simulink model "ammclib_gdflib_iir2_s32k14x"  (Simulink 9.0)
settings: Solver=FixedStepDiscrete  StartTime=0.0  StopTime=5  FixedStep=0.001  RelTol=1e-3  EnableMultiTasking=on
PostLoadFcn:
  | ammclib_gdflib_iir2_s32k14x_params()
InitFcn:
  | mbd_s32k_consistency_checks(bdroot(gcs));
undefined symbols (not defined in the file or in its folder): LQFP
libraries: ammclib_bam_s32k14x x7, mbd_s32k1xx_ec_toolbox x2, simulink x1
Description:
  | This model tests the AMMCLIB GDFLIB IIR2 blocks
  | 
  | Validation:
  | - Run the model in Simulation and check if the results look like the ones shown in the scope capture
  | - Open Freemaster (ammclib_gdflib_iir2_s32k14x.pmp) and compare the HW results against the Simulated ones
CloseFcn:
  | clear all;
settings Model: Creator=NXP MBDT Team  LastModifiedBy=nxf35172
settings DataIOCC: ExternalInput=off  InitialState=off  LimitDataPoints=on  SaveOutput=off  SignalLogging=off  SaveTime=off
settings OptimizationCC: DefaultParameterBehavior=Inlined  LifeSpan=1
settings DebuggingCC: SolverPrmCheckMsg=warning  InheritedTsInSrcMsg=none  SingleTaskRateTransMsg=error  ParameterPrecisionLossMsg=none  UnconnectedInputMsg=error  UnconnectedOutputMsg=error  UnconnectedLineMsg=error  AllowSymbolicDim=off  UnknownTsInhSupMsg=error  StateNameClashWarn=warning
settings HardwareCC: ProdLargestAtomicInteger=Long  ProdLargestAtomicFloat=Double  ProdEndianess=LittleEndian  ProdHWDeviceType=ARM Compatible->ARM Cortex
settings SFSimCC: MATLABDynamicMemAlloc=off
settings RTWCC: SystemTargetFile=mbd_s32k.tlc  MakeCommand=mbd_s32k_make_rtw COPY_MDLREF_INCLUDES=0  TemplateMakefile=mbd_s32k.tmf  Description=Model Based Design Toolbox S32K14x Code Generation Target
settings CodeAppCC: IgnoreCustomStorageClasses=off
settings STFCustomTargetCC: CombineOutputUpdateFcns=on  ERTCustomFileBanners=on  SupportContinuousTime=off  SupportNonInlinedSFcns=off  RemoveResetFunc=on  MATLABClassNameForMDSCustomization=Simulink.SoftwareTarget.ERTCustomization  GRTInterface=off  SystemTargetFile=mbd_s32k14.tlc
settings ERTTargetCC: MultiwordLength=2048  ParMdlRefBuildCompliant=off  CompOptLevelCompliant=off  ConcurrentExecutionCompliant=off  ModelStepFunctionPrototypeControlCompliant=off  CPPClassGenCompliant=off  UseToolchainInfoCompliant=off  InlinedParameterPlacement=NonHierarchical  ERTCustomFileTemplate=example_file_process.tlc  ConvertIfToSwitch=off  SuppressUnreachableDefaultCases=off  MaxIdInt32=IIR2X_int32_T  MaxIdUint32=IIR2X_uint32_T  MaxIdInt16=IIR2X_int16_T  MaxIdUint16=IIR2X_uint16_T  MaxIdInt8=IIR2X_int8_T  MaxIdUint8=IIR2X_uint8_T

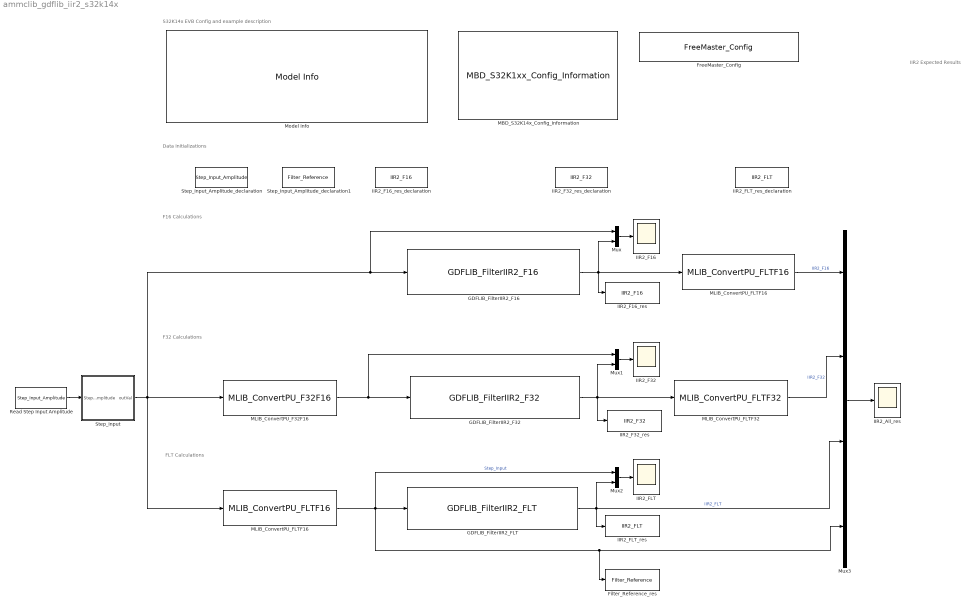
== system ammclib_gdflib_iir2_s32k14x ==
  note: IIR2 Expected Results
  note: S32K14x EVB Config and example description
  note: Data Initializations
  note: F16 Calculations
  note: F32 Calculations
  note: FLT Calculations
  Filter_Reference_res : DataStoreWrite  DataStoreName=Filter_Reference
  FreeMaster_Config : mbd_s32k1xx_ec_toolbox/Utility Blocks/FreeMaster_Config  interface=LPUART1  baudrate=115200  rxd=PTC6: [LPUART1_RX | Receive]  txd=PTC7: [LPUART1_TX | Transmit]  mode=Short Interrupt  isr_prio=15  show_adv_opts=off  use_scope=on  max_scope_vars=8  use_recorder=on  max_rec_vars=8  rec_buff_size=1024  rec_timebase=0 milliseconds  comm_buffer_size_auto=on  comm_buffer_size=255  comm_rqueue_size_default=on  comm_rqueue_size=32
  GDFLIB_FilterIIR2_F16 : ammclib_bam_s32k14x/GDFLIB/bam_f16/GDFLIB_FilterIIR2_F16  f16B0=f16B0  f16B1=f16B1  f16B2=f16B2  f16A1=f16A1  f16A2=f16A2
  GDFLIB_FilterIIR2_F32 : ammclib_bam_s32k14x/GDFLIB/bam_f32/GDFLIB_FilterIIR2_F32  f32B0=f32B0  f32B1=f32B1  f32B2=f32B2  f32A1=f32A1  f32A2=f32A2
  GDFLIB_FilterIIR2_FLT : ammclib_bam_s32k14x/GDFLIB/bam_flt/GDFLIB_FilterIIR2_FLT  fltB0=fltB0  fltB1=fltB1  fltB2=fltB2  fltA1=fltA1  fltA2=fltA2
  IIR2_All_res : Scope
  IIR2_F16 : Scope
  IIR2_F16_res : DataStoreWrite  DataStoreName=IIR2_F16
  IIR2_F16_res_declaration : DataStoreMemory  Priority=2  DataStoreName=IIR2_F16  ReadBeforeWriteMsg=warning  WriteAfterWriteMsg=warning  WriteAfterReadMsg=warning  ShowAdditionalParam=off  OutDataTypeStr=int16
  IIR2_F32 : Scope
  IIR2_F32_res : DataStoreWrite  DataStoreName=IIR2_F32
  IIR2_F32_res_declaration : DataStoreMemory  Priority=2  DataStoreName=IIR2_F32  ReadBeforeWriteMsg=warning  WriteAfterWriteMsg=warning  WriteAfterReadMsg=warning  ShowAdditionalParam=off  OutDataTypeStr=int32
  IIR2_FLT : Scope
  IIR2_FLT_res : DataStoreWrite  DataStoreName=IIR2_FLT
  IIR2_FLT_res_declaration : DataStoreMemory  Priority=2  DataStoreName=IIR2_FLT  ReadBeforeWriteMsg=warning  WriteAfterWriteMsg=warning  WriteAfterReadMsg=warning  ShowAdditionalParam=off  OutDataTypeStr=single
  MBD_S32K14x_Config_Information : mbd_s32k1xx_ec_toolbox/MBD_S32K1xx_Config_Information  Priority=0  mbdt_ver=0  disp_str=|  config_params=[]  mcu_target_name=S32K144  mcu_target_package=100-LQFP  mcu_target_sram_size=64KB  mcu_system_clock_freq=80  mcu_xtal_freq=External 8  mcu_steptick_timer=LPIT Channel 0  mcu_steptick_prio=15  ds_import_enable=on  target_compiler=GCC  target_memory=FLASH  gcc_target_compile_opts=-mcpu=cortex-m4 -mthumb -mfloat-abi=hard -mfpu=fpv4-sp-d16 -O1 -g -gstrict-dwarf  gcc_target_assemble_opts=-mcpu=cortex-m4 -mthumb -mfloat-abi=hard -mfpu=fpv4-sp-d16 -g  gcc_target_link_opts=-mcpu=cortex-m4 -mthumb -mfloat-abi=hard -mfpu=fpv4-sp-d16  gcc_target_default_lcf=on  gcc_target_user_lcf=S32K144_64_flash.ld  ghs_target_compile_opts=-cpu=cortexm4f -thumb -DARM_MATH_CM4 -fpu=vfpv4_d16 -fsingle -Ogeneral -Wundef -Wimplicit-int -Wshadow -Wtrigraphs --no_commons --gnu_asm -gnu99 -gdwarf-2 -G  ghs_target_assemble_opts=-cpu=cortexm4f -fpu=vfpv4_d16  ghs_target_link_opts=-cpu=cortexm4f -thumb -fpu=vfpv4_d16  ghs_target_default_lcf=off  ghs_target_user_lcf=S32K144_64_flash.ld  iar_target_compile_opts=--cpu=Cortex-M4F --thumb --fpu=VFPv4_sp -Ol -e --debug --dlib_config normal  iar_target_assemble_opts=--cpu Cortex-M4F --thumb --fpu VFPv4_sp  iar_target_link_opts=--no_exceptions --vfe --inline  iar_target_default_lcf=off  iar_target_user_lcf=S32K144_64_flash.icf  pil_download_enable=off  rbl_download_enable=on  rbl_start_delay=5000000  rbl_download_interface=OpenSDA  rbl_restart_request=off  rbl_com_port=Custom  rbl_com_port_custom=COM1  pil_download_rate=57600  pil_opensda_drive=Custom  pil_opensda_drive_custom=D  pil_uart_instance=0  pil_uart_rx=PTA2: [LPUART0_RX | Receive]  pil_uart_tx=PTA3: [LPUART0_TX | Transmit]  FTM_PWM_PcrCheckEnDis=on  FTM_Input_Edge_Inputs_PcrCheckEnDis=on  FTM_Dual_Edge_Inputs_PcrCheckEnDis=on  FTM_Quadrature_Inputs_PcrCheckEnDis=on  FTM_Hall_Sensor_Inputs_PcrCheckEnDis=on  LPTMR_PcrCheckEnDis=on  PIT_PcrCheckEnDis=on  RTC_PcrCheckEnDis=on  FlexCAN_PcrCheckEnDis=on  LIN_PcrCheckEnDis=on  FlexIO_PcrCheckEnDis=on  LPI2C_PcrCheckEnDis=on  LPSPI_PcrCheckEnDis=on  LPUART_PcrCheckEnDis=on  CMP_PcrCheckEnDis=on  GPIO_OutputPcrCheckEnDis=on  GPIO_InputPcrCheckEnDis=on  SBC_PcrCheckEnDis=on  AMMCLIB_PcrCheckEnDis=on  FM_PcrCheckEnDis=on  Profile_PcrCheckEnDis=on  ConfigParams_PcrCheckEnDis=on  ModelRef_PcrCheckEnDis=on  PDB0_PcrCheckEnDis=on  CSEc_PcrCheckEnDis=on  eDMA_PcrCheckEnDis=on  ADC_PcrCheckEnDis=on  WDOG_PcrCheckEnDis=on
      | Target : S32K142-16KB_SRAM
      | Package : 100-pin
      | System clock : 80 MHz
      | XTAL clock : External 8 MHz
      | Compiler : GCC
      | Target Type : FLASH
      | Download Code after build : (OpenSDA: E)
      | Step Tick Interrupt Priority : 15
  MLIB_ConvertPU_F32F16 : ammclib_bam_s32k14x/MLIB/bam_f32/MLIB_ConvertPU_F32F16
  MLIB_ConvertPU_FLTF16 : ammclib_bam_s32k14x/MLIB/bam_flt/MLIB_ConvertPU_FLTF16
  "MLIB_ConvertPU_FLTF16   " : ammclib_bam_s32k14x/MLIB/bam_flt/MLIB_ConvertPU_FLTF16
  MLIB_ConvertPU_FLTF32 : ammclib_bam_s32k14x/MLIB/bam_flt/MLIB_ConvertPU_FLTF32
  Model Info : simulink/Model-Wide Utilities/Model Info  Frame=off  DisplayStringWithTags=|  HorizontalTextAlignment=Left  LeftAlignmentValue=0.02
      | Model Name: %<ModelName>
      | 
      | Description: %<Description>
  Mux : Mux  Inputs=2
  Mux1 : Mux  Inputs=2
  Mux2 : Mux  Inputs=2
  Mux3 : Mux
  Read Step Input Amplitude : DataStoreRead  DataStoreName=Step_Input_Amplitude
  Step_Input : Stateflow chart  TreatAsAtomicUnit=on
  Step_Input_Amplitude_declaration : DataStoreMemory  Priority=1  DataStoreName=Step_Input_Amplitude  WriteAfterWriteMsg=warning  WriteAfterReadMsg=warning  InitialValue=32767  ShowAdditionalParam=off  OutMin=-32768  OutMax=32767  OutDataTypeStr=int16
  Step_Input_Amplitude_declaration1 : DataStoreMemory  Priority=1  DataStoreName=Filter_Reference  WriteAfterWriteMsg=warning  WriteAfterReadMsg=warning  ShowAdditionalParam=off  OutMin=-1  OutMax=1  OutDataTypeStr=single
  wires:
  Step_Input/1(outVal) -> MLIB_ConvertPU_F32F16/1, GDFLIB_FilterIIR2_F16/1, Mux/1, MLIB_ConvertPU_FLTF16/1
  GDFLIB_FilterIIR2_F16/1 -> IIR2_F16_res/1, "MLIB_ConvertPU_FLTF16   "/1, Mux/2
  MLIB_ConvertPU_F32F16/1 -> GDFLIB_FilterIIR2_F32/1, Mux1/1
  GDFLIB_FilterIIR2_F32/1 -> Mux1/2, MLIB_ConvertPU_FLTF32/1, IIR2_F32_res/1
  Mux/1 -> IIR2_F16/1
  MLIB_ConvertPU_FLTF16/1 -> GDFLIB_FilterIIR2_FLT/1, Filter_Reference_res/1, Mux3/4, Mux2/1  "Step_Input"
  Mux3/1 -> IIR2_All_res/1
  "MLIB_ConvertPU_FLTF16   "/1 -> Mux3/1  "IIR2_F16"
  MLIB_ConvertPU_FLTF32/1 -> Mux3/2  "IIR2_F32"
  Read Step Input Amplitude/1 -> Step_Input/1(Step_Input_Amplitude)
  Mux1/1 -> IIR2_F32/1
  Mux2/1 -> IIR2_FLT/1
  GDFLIB_FilterIIR2_FLT/1 -> Mux3/3, Mux2/2, IIR2_FLT_res/1  "IIR2_FLT"

== stateflow chart Step_Input ==
  settings: executeAtInitialization=1
  state A
    du:
    outVal = 0;
    cntr=cntr+1;
  state A1
    du:
    outVal = Step_Input_Amplitude;
    cntr=cntr-1;
  (default) -> A : {cntr=0;}
  A1 -> A : [cntr < 2]
  A -> A1 : [cntr > 1000]
  data: cntr local uint32 [0..12] =0; outVal output int16; Step_Input_Amplitude input int16
